simulink model "CSE_Lab3_No1_Diagram"  (R2023b)
settings: Solver=VariableStepAuto  StartTime=0.0  StopTime=20  RelTol=1e-3
values from neighbouring files (symbols this model uses):
  G1_den = [1 0 0]    [CSE_Lab3_No1_Diagram.m]    (also in CSE_Lab3_No1_ReducedBlockDiagram.m; CSE_Lab3_No2_Matlab.m)
  G1_num = [1]    [CSE_Lab3_No1_Diagram.m]    (also in CSE_Lab3_No1_ReducedBlockDiagram.m; CSE_Lab3_No2_Matlab.m = 1)
  G2_den = [1 1]    [CSE_Lab3_No1_Diagram.m]    (also in CSE_Lab3_No1_ReducedBlockDiagram.m; CSE_Lab3_No2_Matlab.m)
  G2_num = [1]    [CSE_Lab3_No1_Diagram.m]    (also in CSE_Lab3_No1_ReducedBlockDiagram.m; CSE_Lab3_No2_Matlab.m = 1)
  G3_den = [1 0]    [CSE_Lab3_No1_Diagram.m]    (also in CSE_Lab3_No1_ReducedBlockDiagram.m; CSE_Lab3_No2_Matlab.m)
  G3_num = [1]    [CSE_Lab3_No1_Diagram.m]    (also in CSE_Lab3_No1_ReducedBlockDiagram.m; CSE_Lab3_No2_Matlab.m = 1)
  H1_den = [1 0]    [CSE_Lab3_No1_Diagram.m]    (also in CSE_Lab3_No1_ReducedBlockDiagram.m; CSE_Lab3_No2_Matlab.m)
  H1_num = [1]    [CSE_Lab3_No1_Diagram.m]    (also in CSE_Lab3_No1_ReducedBlockDiagram.m; CSE_Lab3_No2_Matlab.m = 1)
  H2_den = [1 -1]    [CSE_Lab3_No1_Diagram.m]    (also in CSE_Lab3_No1_ReducedBlockDiagram.m; CSE_Lab3_No2_Matlab.m)
  H2_num = [1]    [CSE_Lab3_No1_Diagram.m]    (also in CSE_Lab3_No1_ReducedBlockDiagram.m; CSE_Lab3_No2_Matlab.m = 1)
  H3_den = [1 -2]    [CSE_Lab3_No1_Diagram.m]    (also in CSE_Lab3_No1_ReducedBlockDiagram.m; CSE_Lab3_No2_Matlab.m)
  H3_num = [1]    [CSE_Lab3_No1_Diagram.m]    (also in CSE_Lab3_No1_ReducedBlockDiagram.m; CSE_Lab3_No2_Matlab.m = 1)
settings Model: Creator=gelibean  LastModifiedBy=gelibean

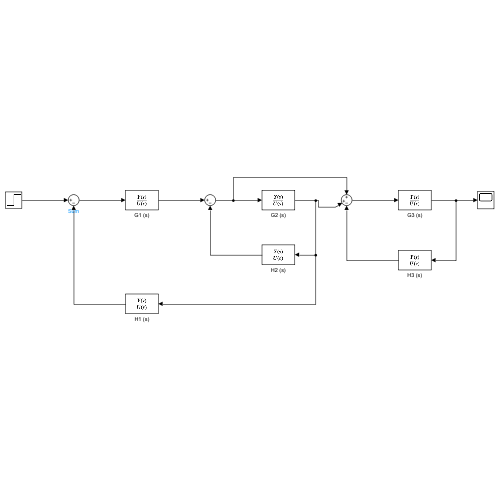
[thumbnail: Simulink's stored preview of the top-level diagram]
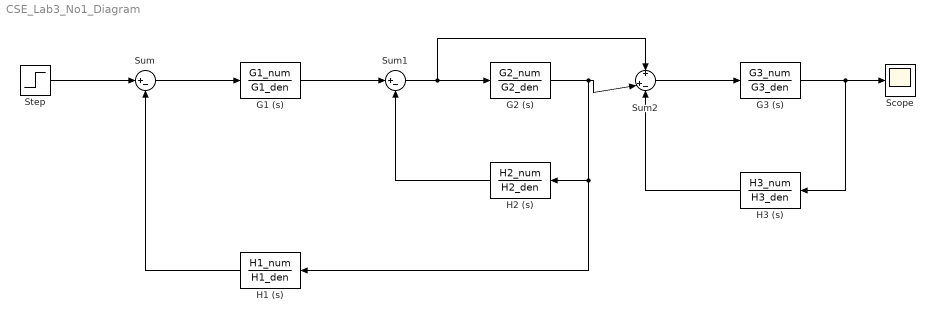
== system CSE_Lab3_No1_Diagram ==
  G1 (s) : TransferFcn  Numerator=G1_num  Denominator=G1_den
  G2 (s) : TransferFcn  Numerator=G2_num  Denominator=G2_den
  G3 (s) : TransferFcn  Numerator=G3_num  Denominator=G3_den
  H1 (s) : TransferFcn  Numerator=H1_num  Denominator=H1_den
  H2 (s) : TransferFcn  Numerator=H2_num  Denominator=H2_den
  H3 (s) : TransferFcn  Numerator=H3_num  Denominator=H3_den
  Scope : Scope
  Step : Step  Time=0  SampleTime=0
  Sum : Sum  Inputs=|+-
  Sum1 : Sum  Inputs=|+-
  Sum2 : Sum  Inputs=+|+-
  wires:
  Step/1 -> Sum/1
  Sum/1 -> G1 (s)/1
  G1 (s)/1 -> Sum1/1
  Sum1/1 -> Sum2/1, G2 (s)/1
  G2 (s)/1 -> H1 (s)/1, H2 (s)/1, Sum2/2
  Sum2/1 -> G3 (s)/1
  G3 (s)/1 -> H3 (s)/1, Scope/1
  H3 (s)/1 -> Sum2/3
  H2 (s)/1 -> Sum1/2
  H1 (s)/1 -> Sum/2
